simulink model "TCP"  (R2015b)
settings: Solver=FixedStepDiscrete  StartTime=0.0  StopTime=100  RelTol=1e-3
undefined symbols (not defined in the file or in its folder): macaddr
libraries: xpcnetworkbufferlib x1, xpcutilitieslib x1, xpcethernetlib x1, instrumentlib x1
settings Model: xpc_rtwmakecfg_data=_xpcnblib_  Creator=Druzhinin_Vasily  LastModifiedBy=Druzhinin_Vasily

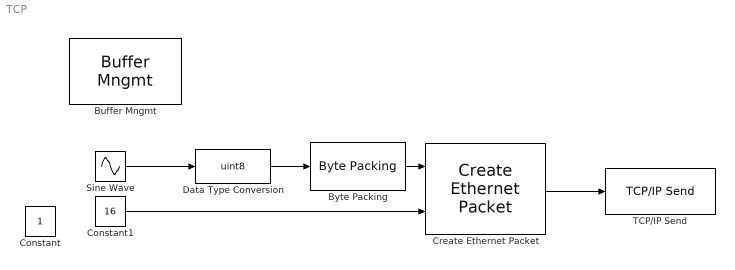
== system TCP ==
  "Buffer Mngmt " : xpcnetworkbufferlib/Buffer Mngmt   Priority=-1  SampleTime=-1  PoolSizes=[100 10 10 200]  ShowTune=on
  "Byte Packing " : xpcutilitieslib/Byte Packing   MaskPackedDataType=double  MaskUnpackedDataTypes={'uint8'}  MaskAlignment=1
  Constant : Constant
  Constant1 : Constant  Value=16
  "Create Ethernet Packet " : xpcethernetlib/Create Ethernet Packet   DstMac=macaddr('00:1B:21:85:37:6C')  EtherType=hex2dec('0000')
  Data Type Conversion : DataTypeConversion  OutDataTypeStr=uint8
  Sine Wave : Sin  SampleTime=0
  TCP/IP Send : instrumentlib/TCP//IP Send  Host=192.168.110.125  Port=11111  EnableBlockingMode=on  Timeout=10  ByteOrder=BigEndian
  wires:
  Data Type Conversion/1 -> "Byte Packing "/1
  "Create Ethernet Packet "/1 -> TCP/IP Send/1
  Constant1/1 -> "Create Ethernet Packet "/2
  "Byte Packing "/1 -> "Create Ethernet Packet "/1
  Sine Wave/1 -> Data Type Conversion/1
